simulink model "sqrt"  (R2021b)
settings: Solver=FixedStepDiscrete  StartTime=0.0  StopTime=0.0002  RelTol=1e-3
model workspace (MAT data in the model file):
  test = 0
undefined symbols (not defined in the file): a, b, c
libraries: hdlsllib x3
settings Model: DataTypeOverride=Off  FPTShortcutValueString='{{},{''BaselineRun'',1,1,1,''BaselineRun'','''',{},''M'',''F'',''''},{''EmbeddedRun'',1,1,1,''EmbeddedRun'','''',{},''M'','''',''''}}'  Creator=max_d  LastModifiedBy=max_d
settings SolverCC: AlgebraicLoopSolver=TrustRegion  AutoInsertRateTranBlk=on
settings DataIOCC: LimitDataPoints=on  SaveOutput=off  SaveTime=off
settings OptimizationCC: BlockReduction=off  ConditionallyExecuteInputs=off  DefaultParameterBehavior=Inlined  InheritOutputTypeSmallerThanSingle=on  LifeSpan=inf
settings DebuggingCC: SignalRangeChecking=warning  AlgebraicLoopMsg=error  SingleTaskRateTransMsg=error  AllowSymbolicDim=off  StrictBusMsg=ErrorOnBusTreatedAsVector  SFUnexpectedBacktrackingDiag=warning  SFNoUnconditionalDefaultTransitionDiag=warning  SFExecutionAtInitializationDiag=none  SFMachineParentedDataDiag=warning  ArithmeticOperatorsInVariantConditions=warning
settings HardwareCC: ProdBitPerPointer=32  ProdBitPerSizeT=32  ProdBitPerPtrDiffT=32  ProdLargestAtomicFloat=None  ProdIntDivRoundTo=Undefined  ProdEndianess=Unspecified  ProdWordSize=32  ProdHWDeviceType=ASIC/FPGA->ASIC/FPGA  ProdEqTarget=off
settings SFSimCC: SimUseLocalCustomCode=off  CustomCodeUndefinedFunction=UseInterfaceOnly
settings RTWCC: RTWUseLocalCustomCode=off
settings CodeAppCC: StateflowObjectComments=on
settings GRTTargetCC: TargetLangStandard=C89/C90 (ANSI)
settings ConfigComp: CovScope=ReferencedModels  CovMetricSettings=dw  CovSaveCumulativeToWorkspaceVar=on  CovSaveSingleToWorkspaceVar=on  CovExternalEMLEnable=off  CovSFcnEnable=off

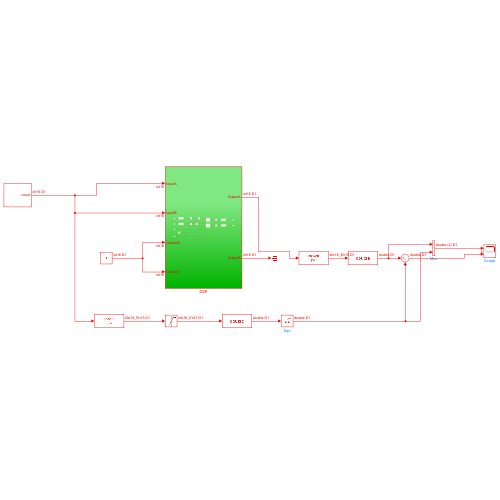
[thumbnail: Simulink's stored preview of the top-level diagram]
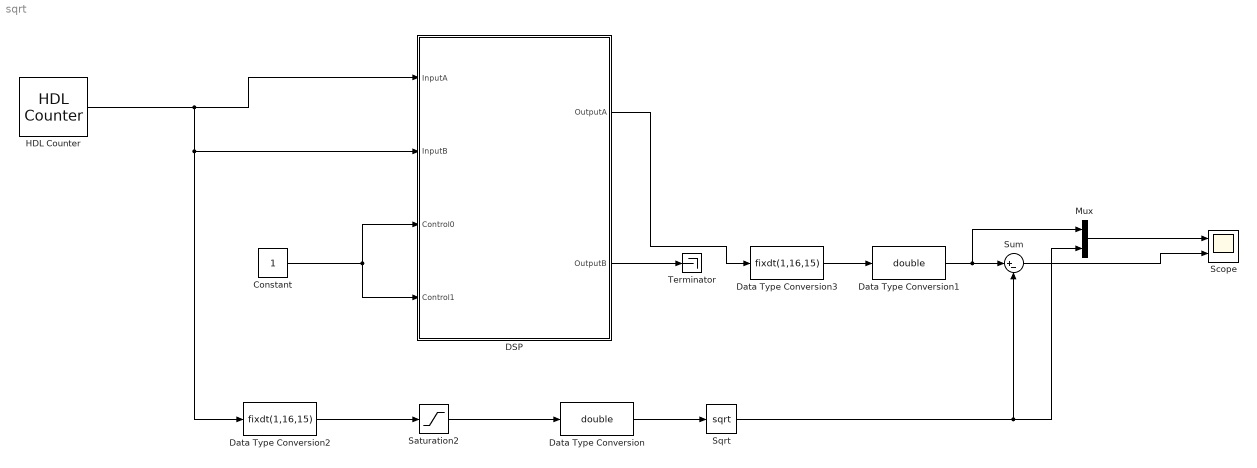
== system sqrt ==
  Constant : Constant  OutDataTypeStr=int16  SampleTime=1/312.5e6
  DSP : Subsystem
  Data Type Conversion : DataTypeConversion  OutDataTypeStr=double
  Data Type Conversion1 : DataTypeConversion  OutDataTypeStr=double
  Data Type Conversion2 : DataTypeConversion  OutDataTypeStr=fixdt(1,16,15)  ConvertRealWorld=Stored Integer (SI)
  Data Type Conversion3 : DataTypeConversion  OutDataTypeStr=fixdt(1,16,15)  ConvertRealWorld=Stored Integer (SI)
  HDL Counter : hdlsllib/Sources/HDL Counter  CountType=Free running  CountInit=0  CountStep=1  CountMax=25  CountFromType=Initial value  CountFrom=0  CountResetPort=off  CountLoadPort=off  CountEnbPort=off  CountDirPort=off  CountHitOutputPort=off  CountDataType=Signed  CountWordLen=16  CountFracLen=0  CountSampTime=1/312.5e6
  Mux : Mux  Inputs=2
  Saturation2 : Saturate  UpperLimit=1  LowerLimit=0
  Scope : Scope  NumInputPorts=2
  Sqrt : Sqrt  SaturateOnIntegerOverflow=on
  Sum : Sum  Inputs=|+-
  Terminator : Terminator
  wires:
  Constant/1 -> DSP/3(Control0), DSP/4(Control1)
  HDL Counter/1 -> Data Type Conversion2/1, DSP/2(InputB), DSP/1(InputA)
  DSP/2(OutputB) -> Terminator/1
  Sqrt/1 -> Mux/2, Sum/2
  Data Type Conversion1/1 -> Mux/1, Sum/1
  Saturation2/1 -> Data Type Conversion/1
  Data Type Conversion/1 -> Sqrt/1
  Data Type Conversion2/1 -> Saturation2/1
  DSP/1(OutputA) -> Data Type Conversion3/1
  Data Type Conversion3/1 -> Data Type Conversion1/1
  Mux/1 -> Scope/1
  Sum/1 -> Scope/2

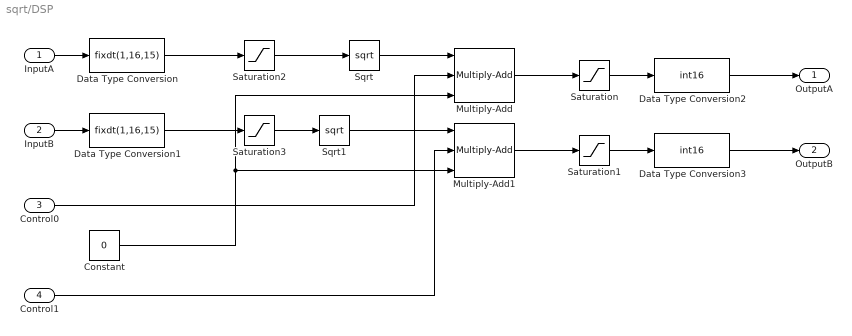
== system sqrt/DSP ==
  InputA : Inport  OutDataTypeStr=fixdt(1,16,0)
  InputB : Inport  Port=2  OutDataTypeStr=fixdt(1,16,0)
  Control0 : Inport  Port=3  OutDataTypeStr=fixdt(1,16,0)
  Control1 : Inport  Port=4  OutDataTypeStr=fixdt(1,16,0)
  Constant : Constant  Value=0  OutDataTypeStr=int16  SampleTime=1/312.5e6
  Data Type Conversion : DataTypeConversion  OutDataTypeStr=fixdt(1,16,15)  ConvertRealWorld=Stored Integer (SI)
  Data Type Conversion1 : DataTypeConversion  OutDataTypeStr=fixdt(1,16,15)  ConvertRealWorld=Stored Integer (SI)
  Data Type Conversion2 : DataTypeConversion  OutDataTypeStr=int16  ConvertRealWorld=Stored Integer (SI)
  Data Type Conversion3 : DataTypeConversion  OutDataTypeStr=int16  ConvertRealWorld=Stored Integer (SI)
  Multiply-Add : hdlsllib/HDL Operations/Multiply-Add  Function=c+(a.*b)  datatype=Inherit: Inherit via internal rule  DoSatur=off  FMA=off
      settings: SourceProductBaseCode=SL
  Multiply-Add1 : hdlsllib/HDL Operations/Multiply-Add  Function=c+(a.*b)  datatype=Inherit: Inherit via internal rule  DoSatur=off  FMA=off
      settings: SourceProductBaseCode=SL
  Saturation : Saturate  UpperLimit=1  LowerLimit=-1
  Saturation1 : Saturate  UpperLimit=1  LowerLimit=-1
  Saturation2 : Saturate  UpperLimit=1  LowerLimit=0
  Saturation3 : Saturate  UpperLimit=1  LowerLimit=0
  Sqrt : Sqrt  OutputSignalType=real  SaturateOnIntegerOverflow=on
  Sqrt1 : Sqrt  OutputSignalType=real  SaturateOnIntegerOverflow=on
  OutputA : Outport  OutDataTypeStr=fixdt(1,16,0)  VectorParamsAs1DForOutWhenUnconnected=off
  OutputB : Outport  Port=2  OutDataTypeStr=fixdt(1,16,0)  VectorParamsAs1DForOutWhenUnconnected=off
  wires:
  Control0/1 -> Multiply-Add/2
  InputA/1 -> Data Type Conversion/1
  InputB/1 -> Data Type Conversion1/1
  Control1/1 -> Multiply-Add1/2
  Constant/1 -> Multiply-Add1/3, Multiply-Add/3
  Multiply-Add/1 -> Saturation/1
  Saturation/1 -> Data Type Conversion2/1
  Multiply-Add1/1 -> Saturation1/1
  Saturation1/1 -> Data Type Conversion3/1
  Data Type Conversion2/1 -> OutputA/1
  Data Type Conversion3/1 -> OutputB/1
  Sqrt/1 -> Multiply-Add/1
  Sqrt1/1 -> Multiply-Add1/1
  Data Type Conversion/1 -> Saturation2/1
  Saturation2/1 -> Sqrt/1
  Data Type Conversion1/1 -> Saturation3/1
  Saturation3/1 -> Sqrt1/1
